simulink model "TD2_Ex1_1_nonlinear"  (R2022a)
settings: Solver=VariableStepAuto  StartTime=0.0  StopTime=20  RelTol=1e-3
undefined symbols (not defined in the file): eps1, eps2, x1e, x2e
settings Model: Creator=CS  LastModifiedBy=CS

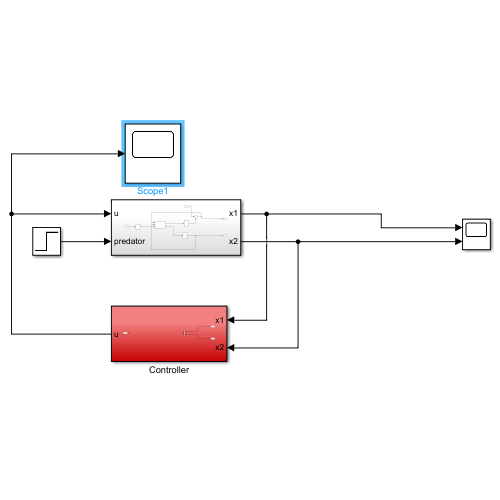
[thumbnail: Simulink's stored preview of the top-level diagram]
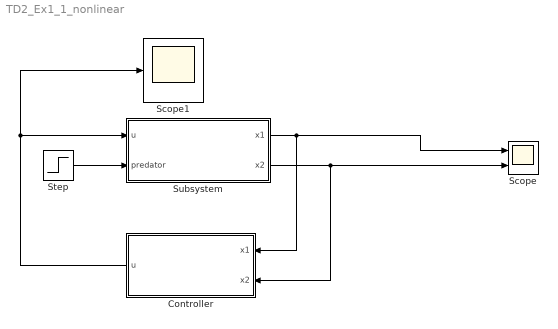
== system TD2_Ex1_1_nonlinear ==
  Controller : Subsystem
  Scope : Scope  NumInputPorts=2
  Scope1 : Scope
  Step : Step  Time=5  After=2  SampleTime=0
  Subsystem : Subsystem
  wires:
  Subsystem/1(x1) -> Controller/1(x1), Scope/1
  Subsystem/2(x2) -> Controller/2(x2), Scope/2
  Step/1 -> Subsystem/2(predator)
  Controller/1(u) -> Scope1/1, Subsystem/1(u)

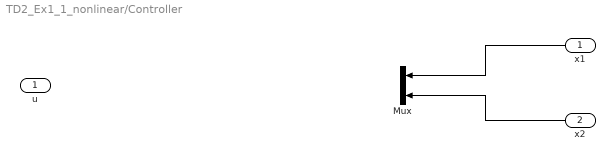
== system TD2_Ex1_1_nonlinear/Controller ==
  x1 : Inport
  x2 : Inport  Port=2
  Mux : Mux  Inputs=2
  u : Outport
  wires:
  x1/1 -> Mux/1
  x2/1 -> Mux/2

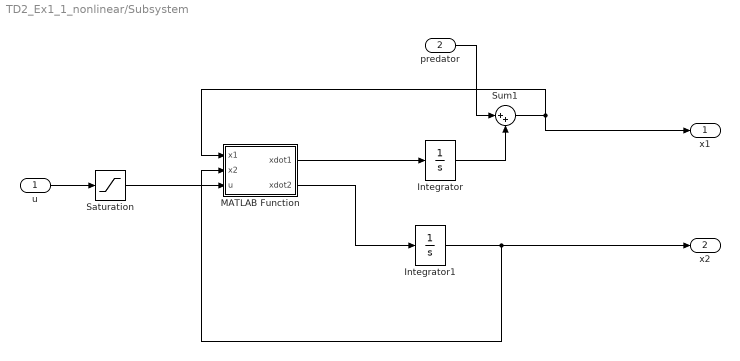
== system TD2_Ex1_1_nonlinear/Subsystem ==
  u : Inport
  predator : Inport  Port=2
  Integrator : Integrator  InitialCondition=x1e+eps1
  Integrator1 : Integrator  InitialCondition=x2e+eps2
  MATLAB Function : MATLAB Function  TreatAsAtomicUnit=on
  Saturation : Saturate  UpperLimit=inf  LowerLimit=0
  Sum1 : Sum  Inputs=|++
  x1 : Outport
  x2 : Outport  Port=2
  wires:
  Integrator1/1 -> MATLAB Function/2(x2), x2/1
  Integrator/1 -> Sum1/2
  Sum1/1 -> x1/1, MATLAB Function/1(x1)
  predator/1 -> Sum1/1
  MATLAB Function/1(xdot1) -> Integrator/1
  u/1 -> Saturation/1
  MATLAB Function/2(xdot2) -> Integrator1/1
  Saturation/1 -> MATLAB Function/3(u)

== matlab function TD2_Ex1_1_nonlinear/Subsystem/MATLAB Function ==
  data: x1 input; x2 input; u input; xdot1 output; xdot2 output
function [xdot1,xdot2] = fcn(x1,x2,u)

xdot1 = -x1+x1*x2;
xdot2 = x2-x1*x2+u;
